simulink model "torqueBalancingSOTSOT2015b86"  (Simulink 8.6)
settings: Solver=FixedStepDiscrete  StartTime=0.0  StopTime="CONFIG.SIMULATION_TIME "  FixedStep=CONFIG.Ts  RelTol=1e-3
InitFcn:
  | cd(fileparts(which(bdroot)));
  | initTorqueBalancingSOT;
undefined symbols (not defined in the file or in its folder): CONFIG, ConstraintsFeetMatrix, gain, references, ROBOT_DOF, ROBOT_DOF_FOR_SIMULINK, sat, SM, sm, upperBoundFeetConstraints, WBT_robotName
libraries: WBToolboxLibrary x135, simulink x8
(part 1 of 3)
settings Model: Creator=daniele  LastModifiedBy=marie
settings DataIOCC: SignalLoggingSaveFormat=Dataset
settings DebuggingCC: FcnCallInpInsideContextMsg=EnableAllAsWarning
settings SFSimCC: SimParseCustomCode=off

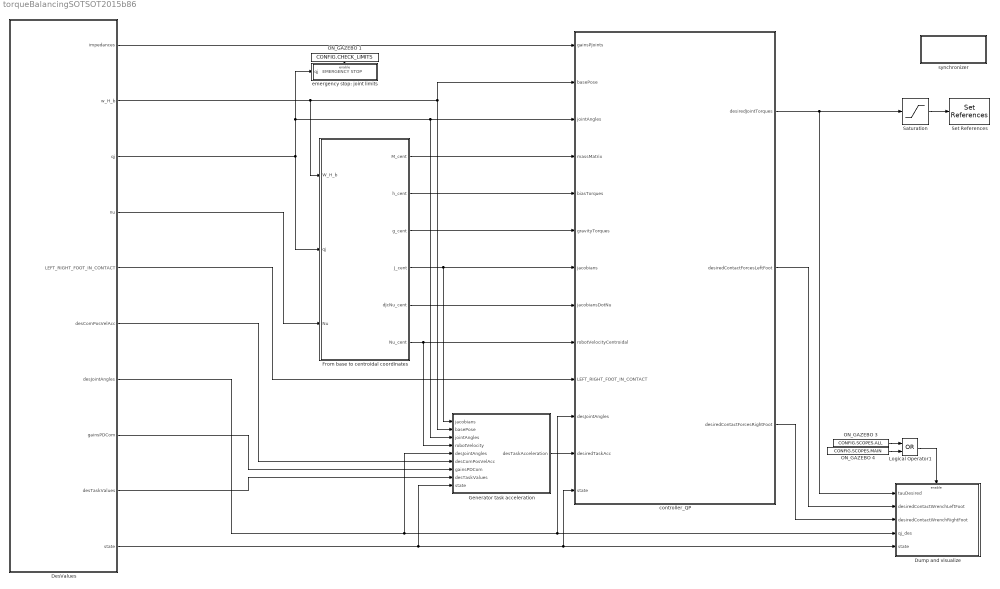
== system torqueBalancingSOTSOT2015b86 ==
  DesValues : Subsystem  Priority=-10
  Dump and visualize : Subsystem
  From base to centroidal coordinates : Subsystem
  Generator task acceleration : Subsystem
  Logical Operator1 : Logic  Operator=OR  AllPortsSameDT=off  OutDataTypeStr=boolean
  ON_GAZEBO 1 : Constant  Value=CONFIG.CHECK_LIMITS
  ON_GAZEBO 3 : Constant  Value=CONFIG.SCOPES.ALL
  ON_GAZEBO 4 : Constant  Value=CONFIG.SCOPES.MAIN
  Saturation : Saturate  UpperLimit=sat.torque  LowerLimit=-sat.torque
  Set References : WBToolboxLibrary/wholeBodyActuators/Set References  controlType=Torque  fullOrSubControl=Full  controlledJoints=''  robotName=WBT_robotName  localName=WBT_modelName  wbiFile=WBT_wbiFilename  wbiList=WBT_wbiList
  controller_QP : Subsystem
  emergency stop: joint limits : Subsystem
  synchronizer : Subsystem
      mask Display: disp('SYNCHRONIZER')
  wires:
  From base to centroidal coordinates/1(M_cent) -> controller_QP/4(massMatrix)
  From base to centroidal coordinates/2(h_cent) -> controller_QP/5(biasTorques)
  controller_QP/1(desiredJointTorques) -> Dump and visualize/1(tauDesired), Saturation/1
  DesValues/7(desJointAngles) -> Dump and visualize/4(qj_des), controller_QP/11(desJointAngles), Generator task acceleration/5(desJointAngles)
  DesValues/5(LEFT_RIGHT_FOOT_IN_CONTACT) -> controller_QP/10(LEFT_RIGHT_FOOT_IN_CONTACT)
  DesValues/6(desComPosVelAcc) -> Generator task acceleration/6(desComPosVelAcc)
  DesValues/1(impedances) -> controller_QP/1(gainsPJoints)
  Saturation/1 -> Set References/1
  DesValues/2(w_H_b) -> From base to centroidal coordinates/1(W_H_b), Generator task acceleration/2(basePose), controller_QP/2(basePose)
  DesValues/4(nu) -> From base to centroidal coordinates/3(Nu)
  Logical Operator1/1 -> Dump and visualize/Enable
  DesValues/10(state) -> Generator task acceleration/9(state), controller_QP/13("state "), Dump and visualize/5(state)
  ON_GAZEBO 1/1 -> emergency stop: joint limits/Enable
  ON_GAZEBO 3/1 -> Logical Operator1/1
  ON_GAZEBO 4/1 -> Logical Operator1/2
  DesValues/3(qj) -> From base to centroidal coordinates/2(qj), emergency stop: joint limits/1(qj   EMERGENCY STOP), Generator task acceleration/3(jointAngles), controller_QP/3(jointAngles)
  From base to centroidal coordinates/3(g_cent) -> controller_QP/6(gravityTorques)
  From base to centroidal coordinates/4(J_cent) -> Generator task acceleration/1(jacobians), controller_QP/7("jacobians ")
  From base to centroidal coordinates/5(dJcNu_cent) -> controller_QP/8(jacobiansDotNu)
  From base to centroidal coordinates/6(Nu_cent) -> Generator task acceleration/4(robotVelocity), controller_QP/9(robotVelocityCentroidal)
  Generator task acceleration/1(desTaskAcceleration) -> controller_QP/12(desiredTaskAcc)
  controller_QP/2(desiredContactForcesLeftFoot) -> Dump and visualize/2(desiredContactWrenchLeftFoot)
  controller_QP/3(desiredContactForcesRightFoot) -> Dump and visualize/3(desiredContactWrenchRightFoot)
  DesValues/8(gainsPDCom) -> Generator task acceleration/7(gainsPDCom)
  DesValues/9(desTaskValues) -> Generator task acceleration/8(desTaskValues)

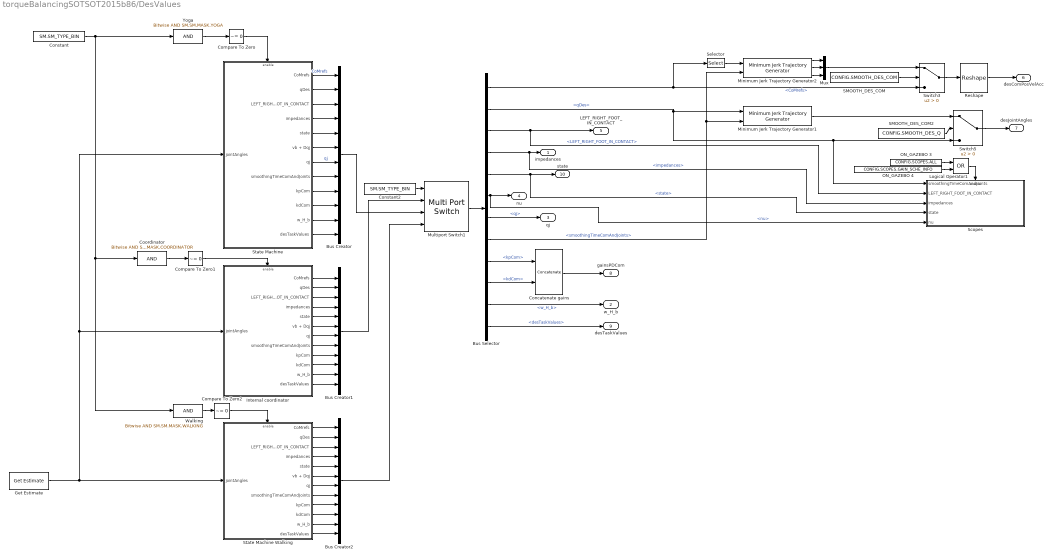
== system torqueBalancingSOTSOT2015b86/DesValues ==
  Bus Creator : BusCreator  Inputs='CoMrefs','qDes','LEFT_RIGHT_FOOT_IN_CONTACT','impedances','state','nu','qj','smoothingTimeComAndJoints','kpCom','kdCom','w_H_b','desTaskValues'
  Bus Creator1 : BusCreator  Inputs='CoMrefs','qDes','LEFT_RIGHT_FOOT_IN_CONTACT','impedances','state','nu','qj','smoothingTimeComAndJoints','kpCom','kdCom','w_H_b','desTaskValues'
  Bus Creator2 : BusCreator  Inputs='CoMrefs','qDes','LEFT_RIGHT_FOOT_IN_CONTACT','impedances','state','nu','qj','smoothingTimeComAndJoints','kpCom','kdCom','w_H_b','desTaskValues'
  Bus Selector : BusSelector  OutputSignals=CoMrefs,qDes,LEFT_RIGHT_FOOT_IN_CONTACT,impedances,state,nu,qj,smoothingTimeComAndJoints,kpCom,kdCom,w_H_b,desTaskValues
  Compare To Zero : simulink/Logic and Bit Operations/Compare To Zero  relop=~=  OutDataTypeStr=boolean
  Compare To Zero1 : simulink/Logic and Bit Operations/Compare To Zero  relop=~=  OutDataTypeStr=boolean
  Compare To Zero2 : simulink/Logic and Bit Operations/Compare To Zero  relop=~=  OutDataTypeStr=boolean
  Concatenate gains : Concatenate  Mode=Multidimensional array  ConcatenateDimension=2
  Constant : Constant  Priority=-10  Value=SM.SM_TYPE_BIN  OutDataTypeStr=uint8
  Constant2 : Constant  Priority=-10  Value=SM.SM_TYPE_BIN  OutDataTypeStr=uint8
  Coordinator : simulink/Logic and Bit Operations/Bitwise Operator  logicop=AND  UseBitMask=on  BitMask=SM.SM.MASK.COORDINATOR  BitMaskRealWorld=Stored Integer
  Get Estimate : WBToolboxLibrary/wholeBodyStates/Get Estimate  estimateType=Joints Position  robotName=WBT_robotName  localName=WBT_modelName  wbiFile=WBT_wbiFilename  wbiList=WBT_wbiList
  Internal coordinator : Subsystem
  Logical Operator1 : Logic  Operator=OR  AllPortsSameDT=off  OutDataTypeStr=boolean
  Minimum Jerk Trajectory Generator1 : WBToolboxLibrary/Utilities/Minimum Jerk Trajectory Generator  externalSettlingTime=on  settlingTime=1  sampleTime=CONFIG.Ts  resetOnSettlingTime=off  firstDerivatives=off  secondDerivatives=off  explicitInitialValue=off
  Minimum Jerk Trajectory Generator2 : WBToolboxLibrary/Utilities/Minimum Jerk Trajectory Generator  externalSettlingTime=on  settlingTime=references.com.smoothingTime  sampleTime=CONFIG.Ts  resetOnSettlingTime=off  firstDerivatives=on  secondDerivatives=on  explicitInitialValue=off
  Multiport Switch1 : MultiPortSwitch  DataPortOrder=Specify indices  DataPortIndices={1, 2, 4}
  Mux : Mux  Inputs=3
  ON_GAZEBO 3 : Constant  Value=CONFIG.SCOPES.ALL
  ON_GAZEBO 4 : Constant  Value=CONFIG.SCOPES.GAIN_SCHE_INFO
  Reshape : Reshape  OutputDimensionality=Customize  OutputDimensions=[3,3]
  SMOOTH_DES_COM : Constant  Value=CONFIG.SMOOTH_DES_COM
  SMOOTH_DES_COM2 : Constant  Value=CONFIG.SMOOTH_DES_Q
  "Scopes  " : Subsystem
  Selector : Selector  InputPortWidth=9  IndexOptions=Index vector (dialog)  Indices=[1 2 3]  OutputSizes=1
  State Machine : Subsystem  Priority=-100
  State Machine Walking : Subsystem  Priority=-100
  Switch3 : Switch  Criteria=u2 > Threshold
  Switch5 : Switch  Criteria=u2 > Threshold
  Walking : simulink/Logic and Bit Operations/Bitwise Operator  logicop=AND  UseBitMask=on  BitMask=SM.SM.MASK.WALKING  BitMaskRealWorld=Stored Integer
  Yoga : simulink/Logic and Bit Operations/Bitwise Operator  logicop=AND  UseBitMask=on  BitMask=SM.SM.MASK.YOGA  BitMaskRealWorld=Stored Integer
  impedances : Outport
  w_H_b : Outport  Port=2
  qj : Outport  Port=3
  nu : Outport  Port=4
  LEFT_RIGHT_FOOT_IN_CONTACT : Outport  Port=5
  desComPosVelAcc : Outport  Port=6
  desJointAngles : Outport  Port=7
  gainsPDCom : Outport  Port=8
  desTaskValues : Outport  Port=9
  state : Outport  Port=10
  wires:
  Reshape/1 -> desComPosVelAcc/1
  Minimum Jerk Trajectory Generator2/1 -> Mux/1
  Minimum Jerk Trajectory Generator2/2 -> Mux/2
  Minimum Jerk Trajectory Generator2/3 -> Mux/3
  Switch3/1 -> Reshape/1
  SMOOTH_DES_COM/1 -> Switch3/2
  SMOOTH_DES_COM2/1 -> Switch5/2
  Switch5/1 -> desJointAngles/1
  State Machine/3(LEFT_RIGHT_FOOT_IN_CONTACT) -> Bus Creator/3
  State Machine/2(qDes) -> Bus Creator/2
  State Machine/1(CoMrefs) -> Bus Creator/1  "CoMrefs"
  State Machine/4(impedances) -> Bus Creator/4
  State Machine/5(state) -> Bus Creator/5
  State Machine/6(vb + Dqj) -> Bus Creator/6
  State Machine/7(qj) -> Bus Creator/7  "qj"
  Bus Selector/7 -> qj/1  "<qj>"
  Yoga/1 -> Compare To Zero/1
  Walking/1 -> Compare To Zero2/1
  Compare To Zero/1 -> State Machine/Enable
  Compare To Zero2/1 -> State Machine Walking/Enable
  Bus Selector/11 -> w_H_b/1  "<w_H_b>"
  Bus Selector/5 -> "Scopes  "/4(state), state/1  "<state>"
  State Machine/8(smoothingTimeComAndJoints) -> Bus Creator/8
  Bus Selector/8 -> Minimum Jerk Trajectory Generator2/2, Minimum Jerk Trajectory Generator1/2  "<smoothingTimeComAndJoints>"
  Logical Operator1/1 -> "Scopes  "/Enable
  Bus Selector/1 -> Selector/1, Switch3/3  "<CoMrefs>"
  Mux/1 -> Switch3/1
  Selector/1 -> Minimum Jerk Trajectory Generator2/1
  Bus Selector/2 -> Minimum Jerk Trajectory Generator1/1, "Scopes  "/1(smoothingTimeComAndJoints), Switch5/3  "<qDes>"
  Minimum Jerk Trajectory Generator1/1 -> Switch5/1
  ON_GAZEBO 3/1 -> Logical Operator1/1
  ON_GAZEBO 4/1 -> Logical Operator1/2
  Bus Selector/6 -> nu/1, "Scopes  "/5(nu)  "<nu>"
  State Machine/9(kpCom) -> Bus Creator/9
  State Machine/10(kdCom) -> Bus Creator/10
  Multiport Switch1/1 -> Bus Selector/1
  Bus Selector/4 -> "Scopes  "/3(impedances), impedances/1  "<impedances>"
  Bus Selector/3 -> "Scopes  "/2(LEFT_RIGHT_FOOT_IN_CONTACT), LEFT_RIGHT_FOOT_IN_CONTACT/1  "<LEFT_RIGHT_FOOT_IN_CONTACT>"
  Constant2/1 -> Multiport Switch1/1
  Concatenate gains/1 -> gainsPDCom/1
  Bus Selector/9 -> Concatenate gains/1  "<kpCom>"
  Bus Selector/10 -> Concatenate gains/2  "<kdCom>"
  Constant/1 -> Walking/1, Coordinator/1, Yoga/1
  Coordinator/1 -> Compare To Zero1/1
  Compare To Zero1/1 -> Internal coordinator/Enable
  Get Estimate/1 -> State Machine Walking/1(jointAngles), State Machine/1(jointAngles), Internal coordinator/1(jointAngles)
  State Machine/11(w_H_b) -> Bus Creator/11
  Bus Creator/1 -> Multiport Switch1/3
  Internal coordinator/1(CoMrefs) -> Bus Creator1/1
  Internal coordinator/2(qDes) -> Bus Creator1/2
  Internal coordinator/3(LEFT_RIGHT_FOOT_IN_CONTACT) -> Bus Creator1/3
  Internal coordinator/4(impedances) -> Bus Creator1/4
  Internal coordinator/5(state) -> Bus Creator1/5
  Internal coordinator/6(vb + Dqj) -> Bus Creator1/6
  Internal coordinator/7(qj) -> Bus Creator1/7
  Internal coordinator/8(smoothingTimeComAndJoints) -> Bus Creator1/8
  Internal coordinator/9(kpCom) -> Bus Creator1/9
  Internal coordinator/10(kdCom) -> Bus Creator1/10
  Internal coordinator/11(w_H_b) -> Bus Creator1/11
  State Machine Walking/1(CoMrefs) -> Bus Creator2/1
  State Machine Walking/2(qDes) -> Bus Creator2/2
  State Machine Walking/3(LEFT_RIGHT_FOOT_IN_CONTACT) -> Bus Creator2/3
  State Machine Walking/4(impedances) -> Bus Creator2/4
  State Machine Walking/5(state) -> Bus Creator2/5
  State Machine Walking/6(vb + Dqj) -> Bus Creator2/6
  State Machine Walking/8(smoothingTimeComAndJoints) -> Bus Creator2/8
  State Machine Walking/9(kpCom) -> Bus Creator2/9
  State Machine Walking/10(kdCom) -> Bus Creator2/10
  State Machine Walking/11(w_H_b) -> Bus Creator2/11
  Bus Creator2/1 -> Multiport Switch1/4
  Bus Creator1/1 -> Multiport Switch1/2
  State Machine/12(desTaskValues) -> Bus Creator/12
  Internal coordinator/12(desTaskValues) -> Bus Creator1/12
  State Machine Walking/12(desTaskValues) -> Bus Creator2/12
  Bus Selector/12 -> desTaskValues/1  "<desTaskValues>"
  State Machine Walking/7(qj) -> Bus Creator2/7

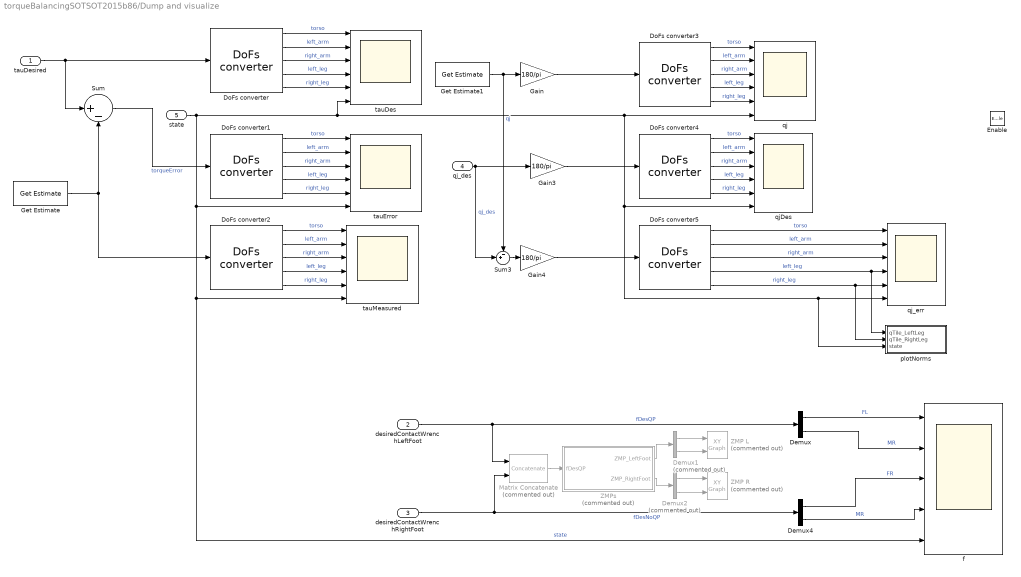
== system torqueBalancingSOTSOT2015b86/Dump and visualize ==
  tauDesired : Inport
  desiredContactWrenchLeftFoot : Inport  Port=2
  desiredContactWrenchRightFoot : Inport  Port=3
  qj_des : Inport  Port=4
  state : Inport  Port=5
  Enable : EnablePort
  Demux : Demux  Outputs=2
  Demux1 : Demux  Commented=on  Outputs=2
  Demux2 : Demux  Commented=on  Outputs=2
  Demux4 : Demux  Outputs=2
  DoFs converter{,1..5} (6 alike) : WBToolboxLibrary/Utilities/DoFs converter  yarp2WBIOption=From WBI to YARP  robotName=WBT_robotName  localName=WBT_modelName  wbiFile=WBT_wbiFilename  wbiList=WBT_wbiList
  Gain : Gain  Gain=180/pi
  Gain3 : Gain  Gain=180/pi
  Gain4 : Gain  Gain=180/pi
  Get Estimate : WBToolboxLibrary/wholeBodyStates/Get Estimate  estimateType=Joints Torque  robotName=WBT_robotName  localName=WBT_modelName  wbiFile=WBT_wbiFilename  wbiList=WBT_wbiList
  Get Estimate1 : WBToolboxLibrary/wholeBodyStates/Get Estimate  estimateType=Joints Position  robotName=WBT_robotName  localName=WBT_modelName  wbiFile=WBT_wbiFilename  wbiList=WBT_wbiList
  Matrix Concatenate : Concatenate  Commented=on  Mode=Multidimensional array
  Sum : Sum  Inputs=|+-
  Sum3 : Sum  Inputs=-+|
  ZMP L : simulink/Sinks/XY Graph  Commented=on  xmin=gain.footSize(1,1)  xmax=gain.footSize(1,2)  ymin=gain.footSize(2,1)  ymax=gain.footSize(2,2)  st=-1
  ZMP R : simulink/Sinks/XY Graph  Commented=on  xmin=gain.footSize(1,1)  xmax=gain.footSize(1,2)  ymin=gain.footSize(2,1)  ymax=gain.footSize(2,2)  st=-1
  ZMPs : Subsystem  Commented=on
  f : Scope  NumInputPorts=5
  plotNorms : Subsystem
  qj : Scope  NumInputPorts=6
  qjDes : Scope  NumInputPorts=6
  qj_err : Scope  NumInputPorts=6
  tauDes : Scope  NumInputPorts=6
  tauError : Scope  NumInputPorts=6
  tauMeasured : Scope  NumInputPorts=6
  wires:
  Get Estimate1/1 -> Sum3/1, Gain/1  "qj"
  Gain/1 -> DoFs converter3/1
  DoFs converter3/5 -> qj/5  "right_leg"
  DoFs converter3/1 -> qj/1  "torso"
  DoFs converter3/2 -> qj/2  "left_arm"
  DoFs converter3/4 -> qj/4  "left_leg"
  DoFs converter3/3 -> qj/3  "right_arm"
  desiredContactWrenchLeftFoot/1 -> Matrix Concatenate/1, Demux/1  "fDesQP"
  ZMPs/1(ZMP_LeftFoot) -> Demux1/1
  ZMPs/2(ZMP_RightFoot) -> Demux2/1
  Demux1/1 -> ZMP L/1
  Demux1/2 -> ZMP L/2
  Demux2/1 -> ZMP R/1
  Demux2/2 -> ZMP R/2
  desiredContactWrenchRightFoot/1 -> Matrix Concatenate/2, Demux4/1  "fDesNoQP"
  tauDesired/1 -> DoFs converter/1, Sum/1
  Get Estimate/1 -> DoFs converter2/1, Sum/2
  DoFs converter/5 -> tauDes/5  "right_leg"
  DoFs converter/1 -> tauDes/1  "torso"
  DoFs converter/2 -> tauDes/2  "left_arm"
  DoFs converter/4 -> tauDes/4  "left_leg"
  DoFs converter/3 -> tauDes/3  "right_arm"
  DoFs converter1/5 -> tauError/5  "right_leg"
  DoFs converter1/1 -> tauError/1  "torso"
  DoFs converter1/2 -> tauError/2  "left_arm"
  DoFs converter1/4 -> tauError/4  "left_leg"
  DoFs converter1/3 -> tauError/3  "right_arm"
  Sum/1 -> DoFs converter1/1  "torqueError"
  DoFs converter2/5 -> tauMeasured/5  "right_leg"
  DoFs converter2/1 -> tauMeasured/1  "torso"
  DoFs converter2/2 -> tauMeasured/2  "left_arm"
  DoFs converter2/4 -> tauMeasured/4  "left_leg"
  DoFs converter2/3 -> tauMeasured/3  "right_arm"
  qj_des/1 -> Sum3/2, Gain3/1  "qj_des"
  Gain3/1 -> DoFs converter4/1
  DoFs converter4/5 -> qjDes/5  "right_leg"
  DoFs converter4/1 -> qjDes/1  "torso"
  DoFs converter4/2 -> qjDes/2  "left_arm"
  DoFs converter4/4 -> qjDes/4  "left_leg"
  DoFs converter4/3 -> qjDes/3  "right_arm"
  Gain4/1 -> DoFs converter5/1
  DoFs converter5/5 -> plotNorms/2(qTile_RightLeg), qj_err/5  "right_leg"
  DoFs converter5/1 -> qj_err/1  "torso"
  DoFs converter5/2 -> qj_err/2  "left_arm"
  DoFs converter5/4 -> plotNorms/1(qTile_LeftLeg), qj_err/4  "left_leg"
  DoFs converter5/3 -> qj_err/3  "right_arm"
  Sum3/1 -> Gain4/1
  state/1 -> tauDes/6, plotNorms/3(state), qj_err/6, qjDes/6, qj/6, f/5, tauMeasured/6, tauError/6  "state"
  Demux/1 -> f/1  "FL"
  Demux/2 -> f/2  "MR"
  Demux4/1 -> f/3  "FR"
  Demux4/2 -> f/4  "MR"
  Matrix Concatenate/1 -> ZMPs/1(fDesQP)

== system torqueBalancingSOTSOT2015b86/From base to centroidal coordinates ==
  W_H_b : Inport
  qj : Inport  Port=2
  Nu : Inport  Port=3
  Centroidal tranformation : Subsystem
  CoM and Base Kinematics : Subsystem
  Jacobians : Subsystem
  Switch{1..6} (6 alike) : Switch  Criteria=u2 > Threshold
  System Dynamics : Subsystem
  USE_IMU4EST_BASE{,1..5} (6 alike) : Constant  Value=CONFIG.USE_CENTROIDALDYN
  M_cent : Outport
  h_cent : Outport  Port=2
  g_cent : Outport  Port=3
  J_cent : Outport  Port=4
  dJcNu_cent : Outport  Port=5
  Nu_cent : Outport  Port=6
  wires:
  Jacobians/2(dJNu) -> Switch4/3, Centroidal tranformation/10(dJcNu)
  System Dynamics/1(h) -> Switch1/3, Centroidal tranformation/2(h)
  System Dynamics/2(g) -> Switch2/3, Centroidal tranformation/3(g)
  System Dynamics/3(M) -> Switch6/3, Centroidal tranformation/4(M)
  CoM and Base Kinematics/1(dx_b) -> Centroidal tranformation/6(dx_b)
  CoM and Base Kinematics/2(xCoM) -> Centroidal tranformation/7(xCoM)
  CoM and Base Kinematics/3(dxCoM) -> Centroidal tranformation/8(dxCoM)
  Jacobians/1(J) -> Switch3/3, Centroidal tranformation/9(Jc)
  qj/1 -> CoM and Base Kinematics/2(qj), System Dynamics/2(qj), Jacobians/2(qj)
  Nu/1 -> Jacobians/3(Nu), CoM and Base Kinematics/3(Nu), Switch5/3, Centroidal tranformation/5(Nu), System Dynamics/3(Nu)
  W_H_b/1 -> Centroidal tranformation/1(w_H_b), Jacobians/1(W_H_b), System Dynamics/1(W_H_b), CoM and Base Kinematics/1(W_H_b)
  USE_IMU4EST_BASE/1 -> Switch6/2
  Switch6/1 -> M_cent/1
  Centroidal tranformation/1(M_centr) -> Switch6/1
  USE_IMU4EST_BASE1/1 -> Switch1/2
  USE_IMU4EST_BASE2/1 -> Switch2/2
  USE_IMU4EST_BASE3/1 -> Switch3/2
  USE_IMU4EST_BASE4/1 -> Switch4/2
  USE_IMU4EST_BASE5/1 -> Switch5/2
  Centroidal tranformation/2(h_centr) -> Switch1/1
  Switch1/1 -> h_cent/1
  Centroidal tranformation/3(g_centr) -> Switch2/1
  Centroidal tranformation/4(Jc_centr) -> Switch3/1
  Switch2/1 -> g_cent/1
  Switch3/1 -> J_cent/1
  Centroidal tranformation/5(dJcNu_centr) -> Switch4/1
  Switch4/1 -> dJcNu_cent/1
  Switch5/1 -> Nu_cent/1
  Centroidal tranformation/6(Nu_centr) -> Switch5/1

== system torqueBalancingSOTSOT2015b86/Generator task acceleration ==
  jacobians : Inport
  basePose : Inport  Port=2
  jointAngles : Inport  Port=3
  robotVelocity : Inport  Port=4
  desJointAngles : Inport  Port=5
  desComPosVelAcc : Inport  Port=6
  gainsPDCom : Inport  Port=7
  desTaskValues : Inport  Port=8
  state : Inport  Port=9
  Bus Selector : BusSelector  OutputSignals=desRootRotPosVelAcc,desLFootRotPosVelAcc,desLFootOriginPosVelAcc,desRFootRotPosVelAcc,desRFootOriginPosVelAcc
  Dump and visualize : Subsystem
  Logical Operator1 : Logic  Operator=OR  AllPortsSameDT=off  OutDataTypeStr=boolean
  ON_GAZEBO 3 : Constant  Value=CONFIG.SCOPES.ALL
  ON_GAZEBO 4 : Constant  Value=CONFIG.SCOPES.MAIN
  Product : Product  Multiplication=Matrix(*)
  desiredTaskAcceleration : MATLAB Function  TreatAsAtomicUnit=on
      settings: PermitHierarchicalResolution=ParametersOnly
  fromDesiredJointAngles to  desRootRotPosVelAcc3 : Subsystem
  leftFootPose : WBToolboxLibrary/wholeBodyModel/Kinematics/Forward Kinematics  frameName='l_sole'  robotName=WBT_robotName  localName=WBT_modelName  wbiFile=WBT_wbiFilename  wbiList=WBT_wbiList
  rightFootPose : WBToolboxLibrary/wholeBodyModel/Kinematics/Forward Kinematics  frameName='r_sole'  robotName=WBT_robotName  localName=WBT_modelName  wbiFile=WBT_wbiFilename  wbiList=WBT_wbiList
  xCom : Subsystem
  desTaskAcceleration : Outport
  wires:
  desiredTaskAcceleration/1(desiredTaskAcc) -> desTaskAcceleration/1
  jointAngles/1 -> rightFootPose/2, leftFootPose/2, xCom/2(qj)
  robotVelocity/1 -> Product/2
  basePose/1 -> rightFootPose/1, leftFootPose/1, xCom/1(w_H_b)
  jacobians/1 -> Product/1
  desJointAngles/1 -> fromDesiredJointAngles to  desRootRotPosVelAcc3/1(desJointAngles)
  xCom/1(xCom) -> desiredTaskAcceleration/1(comPos)
  fromDesiredJointAngles to  desRootRotPosVelAcc3/1(fixed_link_R_root) -> desiredTaskAcceleration/3(w_R_root)
  desComPosVelAcc/1 -> desiredTaskAcceleration/2(desComPosVelAcc), Dump and visualize/3(comDes)
  leftFootPose/1 -> desiredTaskAcceleration/5(w_H_l_sole)
  Bus Selector/2 -> Dump and visualize/8(desLFootRot), desiredTaskAcceleration/6(desLFootRotPosVelAcc)  "<desLFootRotPosVelAcc>"
  Product/1 -> desiredTaskAcceleration/11(taskVelocities)
  gainsPDCom/1 -> desiredTaskAcceleration/12(gainsPDCom)
  Bus Selector/1 -> desiredTaskAcceleration/4(desRootRotPosVelAcc), Dump and visualize/1(desRootRot)  "<desRootRotPosVelAcc>"
  Bus Selector/3 -> desiredTaskAcceleration/7(desLFootOriginPosVelAcc), Dump and visualize/6(desLFootPos)  "<desLFootOriginPosVelAcc>"
  rightFootPose/1 -> desiredTaskAcceleration/8(w_H_r_sole)
  Bus Selector/4 -> desiredTaskAcceleration/9(desRFootRotPosVelAcc), Dump and visualize/12(desRFootRot)  "<desRFootRotPosVelAcc>"
  Bus Selector/5 -> desiredTaskAcceleration/10(desRFootOriginPosVelAcc), Dump and visualize/10(desRFootPos)  "<desRFootOriginPosVelAcc>"
  Logical Operator1/1 -> Dump and visualize/Enable
  ON_GAZEBO 3/1 -> Logical Operator1/1
  ON_GAZEBO 4/1 -> Logical Operator1/2
  desiredTaskAcceleration/2(comError) -> Dump and visualize/2(comErr)
  desiredTaskAcceleration/3(rootRotErr) -> Dump and visualize/4(rootRotErr)
  desiredTaskAcceleration/4(lFootPosErr) -> Dump and visualize/5(lFootPosErr)
  desiredTaskAcceleration/5(lFootRotErr) -> Dump and visualize/7(lFoorRotErr)
  desiredTaskAcceleration/6(rFootPosErr) -> Dump and visualize/9(rFootPosErr)
  desiredTaskAcceleration/7(rFootRotErr) -> Dump and visualize/11(rFoorRotErr)
  state/1 -> Dump and visualize/13(state), fromDesiredJointAngles to  desRootRotPosVelAcc3/2(state)
  desTaskValues/1 -> Bus Selector/1

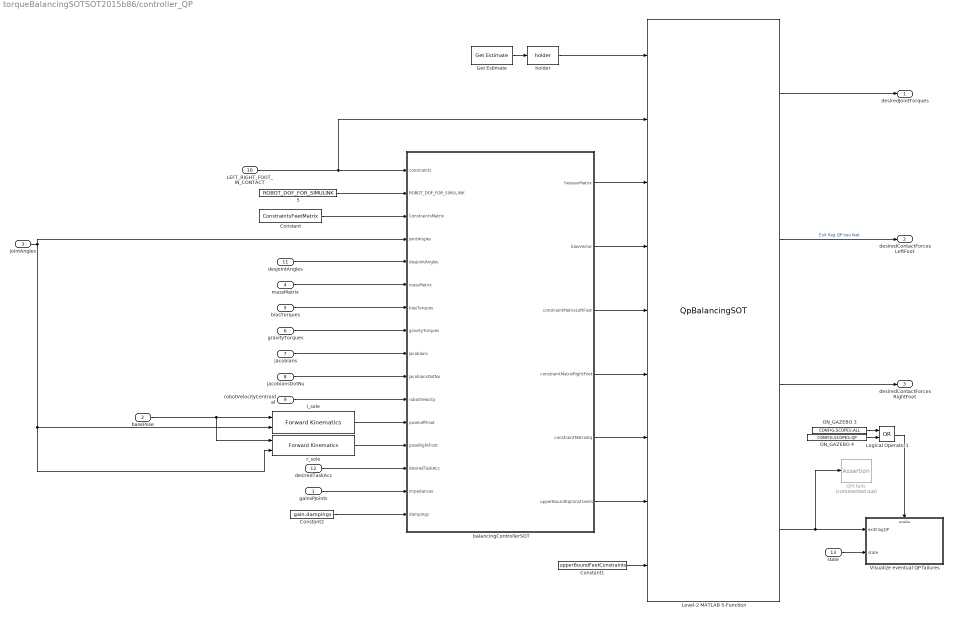
== system torqueBalancingSOTSOT2015b86/controller_QP ==
  gainsPJoints : Inport
  basePose : Inport  Port=2
  jointAngles : Inport  Port=3
  massMatrix : Inport  Port=4
  biasTorques : Inport  Port=5
  gravityTorques : Inport  Port=6
  "jacobians " : Inport  Port=7
  jacobiansDotNu : Inport  Port=8
  robotVelocityCentroidal : Inport  Port=9
  LEFT_RIGHT_FOOT_IN_CONTACT : Inport  Port=10
  desJointAngles : Inport  Port=11
  desiredTaskAcc : Inport  Port=12
  "state " : Inport  Port=13
  "    5" : Constant  Value=ROBOT_DOF_FOR_SIMULINK
  Constant : Constant  Value=ConstraintsFeetMatrix
  Constant1 : Constant  Value=upperBoundFeetConstraints
  Constant2 : Constant  Value=gain.dampings
  Get Estimate : WBToolboxLibrary/wholeBodyStates/Get Estimate  estimateType=Joints Torque  robotName=WBT_robotName  localName=WBT_modelName  wbiFile=WBT_wbiFilename  wbiList=WBT_wbiList
  Level-2 MATLAB S-Function : M-S-Function  FunctionName=QpBalancingSOT  Parameters=ROBOT_DOF,sat.torqueDot,CONFIG.Ts,CONFIG.QP.USE_CONTINUITY_CONSTRAINTS,CONFIG.QP.USE_STRICT_TASK_PRIORITIES  mask{robotDofs=ROBOT_DOF, tauDotMax=sat.torqueDot, Ts=CONFIG.Ts}
      mask prompts: robotDofs "Robt degrees of freedom"; tauDotMax "Maximum derivative of torques"; Ts "Controller period"
      mask Display: disp('QP')
  Logical Operator1 : Logic  Operator=OR  AllPortsSameDT=off  OutDataTypeStr=boolean
  ON_GAZEBO 3 : Constant  Value=CONFIG.SCOPES.ALL
  ON_GAZEBO 4 : Constant  Value=CONFIG.SCOPES.QP
  QPt fails : Assertion  Commented=on
  Visualize eventual QP failures : Subsystem
  balancingControllerSOT : MATLAB Function  TreatAsAtomicUnit=on
      settings: PermitHierarchicalResolution=ParametersOnly
  "holder " : WBToolboxLibrary/Utilities/holder 
  l_sole : WBToolboxLibrary/wholeBodyModel/Kinematics/Forward Kinematics  frameName='l_sole'  robotName=WBT_robotName  localName=WBT_modelName  wbiFile=WBT_wbiFilename  wbiList=WBT_wbiList
  r_sole : WBToolboxLibrary/wholeBodyModel/Kinematics/Forward Kinematics  frameName='r_sole'  robotName=WBT_robotName  localName=WBT_modelName  wbiFile=WBT_wbiFilename  wbiList=WBT_wbiList
  desiredJointTorques : Outport
  desiredContactForcesLeftFoot : Outport  Port=2
  desiredContactForcesRightFoot : Outport  Port=3
  wires:
  jointAngles/1 -> r_sole/2, l_sole/2, balancingControllerSOT/4(jointAngles)
  desJointAngles/1 -> balancingControllerSOT/5(desJointAngles)
  gainsPJoints/1 -> balancingControllerSOT/15(impedances)
  "    5"/1 -> balancingControllerSOT/2(ROBOT_DOF_FOR_SIMULINK)
  Constant/1 -> balancingControllerSOT/3(ConstraintsMatrix)
  Constant1/1 -> Level-2 MATLAB S-Function/9
  basePose/1 -> r_sole/1, l_sole/1
  desiredTaskAcc/1 -> balancingControllerSOT/14(desiredTaskAcc)
  r_sole/1 -> balancingControllerSOT/13(poseRightFoot)
  l_sole/1 -> balancingControllerSOT/12(poseLeftFoot)
  robotVelocityCentroidal/1 -> balancingControllerSOT/11(robotVelocity)
  gravityTorques/1 -> balancingControllerSOT/8(gravityTorques)
  biasTorques/1 -> balancingControllerSOT/7(biasTorques)
  massMatrix/1 -> balancingControllerSOT/6(massMatrix)
  Logical Operator1/1 -> Visualize eventual QP failures/Enable
  LEFT_RIGHT_FOOT_IN_CONTACT/1 -> Level-2 MATLAB S-Function/2, balancingControllerSOT/1(constraints)
  ON_GAZEBO 3/1 -> Logical Operator1/1
  ON_GAZEBO 4/1 -> Logical Operator1/2
  balancingControllerSOT/1(hessianMatrix) -> Level-2 MATLAB S-Function/3
  balancingControllerSOT/2(biasVector) -> Level-2 MATLAB S-Function/4
  balancingControllerSOT/3(constraintMatrixLeftFoot) -> Level-2 MATLAB S-Function/5
  balancingControllerSOT/4(constraintMatrixRightFoot) -> Level-2 MATLAB S-Function/6
  "jacobians "/1 -> balancingControllerSOT/9(jacobians)
  jacobiansDotNu/1 -> balancingControllerSOT/10(jacobiansDotNu)
  Level-2 MATLAB S-Function/1 -> desiredJointTorques/1
  balancingControllerSOT/6(upperBoundEqConstraints) -> Level-2 MATLAB S-Function/8
  balancingControllerSOT/5(constraintMatrixEq) -> Level-2 MATLAB S-Function/7
  Level-2 MATLAB S-Function/3 -> desiredContactForcesRightFoot/1
  Level-2 MATLAB S-Function/2 -> desiredContactForcesLeftFoot/1  "Exit flag QP two feet"
  "state "/1 -> Visualize eventual QP failures/2(state)
  Level-2 MATLAB S-Function/4 -> QPt fails/1, Visualize eventual QP failures/1(exitFlagQP)
  Constant2/1 -> balancingControllerSOT/16(dampings)
  Get Estimate/1 -> "holder "/1
  "holder "/1 -> Level-2 MATLAB S-Function/1

== system torqueBalancingSOTSOT2015b86/emergency stop: joint limits ==
  qj   EMERGENCY STOP : Inport
  Enable : EnablePort
  Assertion : Assertion
  Get Limits : WBToolboxLibrary/wholeBodyStates/Get Limits  limitsType=Position  robotName=WBT_robotName  localName=WBT_modelName  wbiFile=WBT_wbiFilename  wbiList=WBT_wbiList
  MATLAB Function : MATLAB Function  TreatAsAtomicUnit=on
      settings: PermitHierarchicalResolution=ParametersOnly
  index1 : Constant  Value=0.01  VectorParams1D=off
  wires:
  Get Limits/1 -> MATLAB Function/1(umin)
  Get Limits/2 -> MATLAB Function/2(umax)
  index1/1 -> MATLAB Function/4(tol)
  qj   EMERGENCY STOP/1 -> MATLAB Function/3(u)
  MATLAB Function/1(inRange) -> Assertion/1

== system torqueBalancingSOTSOT2015b86/synchronizer ==
  GAZEBO_SYNCHRONIZER : Subsystem
  Logical Operator : Logic  Operator=NOT  AllPortsSameDT=off  OutDataTypeStr=boolean
  "ON_GAZEBO " : Constant  Value=CONFIG.ON_GAZEBO
  REAL_TIME_SYNC : Subsystem
  wires:
  Logical Operator/1 -> REAL_TIME_SYNC/Enable
  "ON_GAZEBO "/1 -> GAZEBO_SYNCHRONIZER/Enable, Logical Operator/1

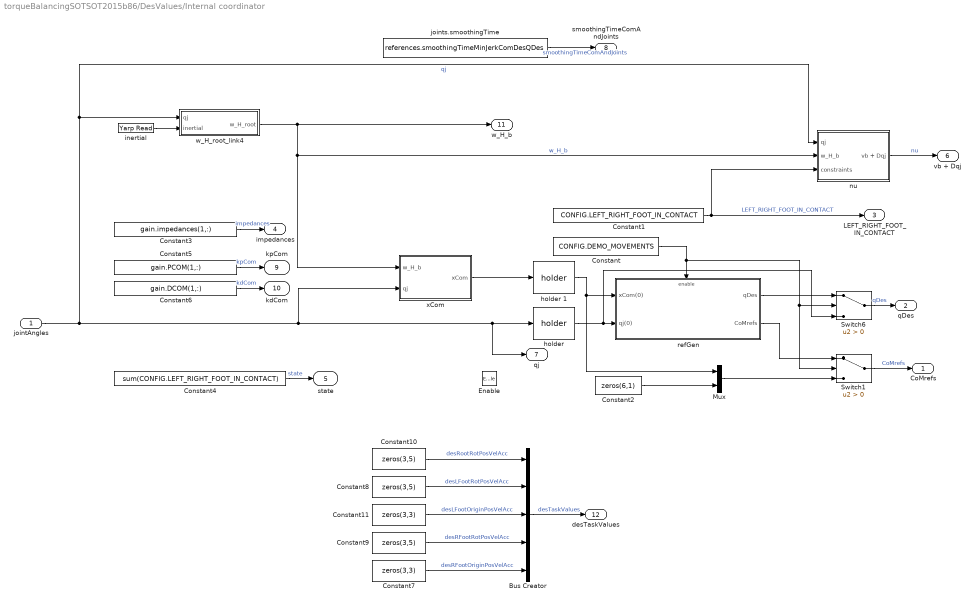
== system torqueBalancingSOTSOT2015b86/DesValues/Internal coordinator ==
  jointAngles : Inport
  Enable : EnablePort
  Bus Creator : BusCreator  Inputs='desRootRotPosVelAcc','desLFootRotPosVelAcc','desLFootOriginPosVelAcc','desRFootRotPosVelAcc','desRFootOriginPosVelAcc'
  Constant : Constant  Value=CONFIG.DEMO_MOVEMENTS
  Constant1 : Constant  Value=CONFIG.LEFT_RIGHT_FOOT_IN_CONTACT
  Constant10 : Constant  Value=zeros(3,5)
  Constant11 : Constant  Value=zeros(3,3)
  Constant2 : Constant  Value=zeros(6,1)
  Constant3 : Constant  Value=gain.impedances(1,:)
  Constant4 : Constant  Value=sum(CONFIG.LEFT_RIGHT_FOOT_IN_CONTACT)
  Constant5 : Constant  Value=gain.PCOM(1,:)
  Constant6 : Constant  Value=gain.DCOM(1,:)
  Constant7 : Constant  Value=zeros(3,3)
  Constant8 : Constant  Value=zeros(3,5)
  Constant9 : Constant  Value=zeros(3,5)
  Mux : Mux  Inputs=2
  Switch1 : Switch  Criteria=u2 > Threshold
  Switch6 : Switch  Criteria=u2 > Threshold
  "holder " : WBToolboxLibrary/Utilities/holder 
  holder 1 : WBToolboxLibrary/Utilities/holder 
  inertial : WBToolboxLibrary/Utilities/Yarp Read  portName=PORTS.IMU  signalSize=12  blocking=off  timestamp=off  autoconnect=on  errorOnConnection=on
  joints.smoothingTime : Constant  Value=references.smoothingTimeMinJerkComDesQDes
  nu : Subsystem
  refGen : Subsystem
  w_H_root_link4 : Subsystem  mask{link_name='l_sole'}
      mask prompts: link_name "link name"
      mask help:
      | This block evaluates the homogeneous transformation between the world and the root link, i.e. ^wH_b. It assumes that the link specified by the variable 'link_name' has a constant position
      | w.r.t. an inertial frame, but it can rotate arbitrarily. This rotation is retrived from the IMU sensor.
      mask Display:
      | str = strrep(link_name, '_','\_');
      | port_label('output',1,['{}^{',str '}H_{root}'],'texmode','on')
      | clear str;
      | 
      | port_label('input',1,'q_j','texmode','on')
      | 
      | port_label('input',2,'inertial','texmode','on')
  xCom : Subsystem
  CoMrefs : Outport
  qDes : Outport  Port=2
  LEFT_RIGHT_FOOT_IN_CONTACT : Outport  Port=3
  impedances : Outport  Port=4
  state : Outport  Port=5
  vb + Dqj : Outport  Port=6
  qj : Outport  Port=7
  smoothingTimeComAndJoints : Outport  Port=8
  kpCom : Outport  Port=9
  kdCom : Outport  Port=10
  w_H_b : Outport  Port=11
  desTaskValues : Outport  Port=12
  wires:
  Constant1/1 -> nu/3("constraints "), LEFT_RIGHT_FOOT_IN_CONTACT/1  "LEFT_RIGHT_FOOT_IN_CONTACT"
  "holder "/1 -> Switch6/3, refGen/2(qj(0))
  Constant/1 -> Switch1/2, Switch6/2, refGen/Enable
  Switch6/1 -> qDes/1  "qDes"
  Switch1/1 -> CoMrefs/1  "CoMrefs"
  refGen/1(qDes) -> Switch6/1
  refGen/2(CoMrefs) -> Switch1/1
  Mux/1 -> Switch1/3
  Constant2/1 -> Mux/2
  Constant3/1 -> impedances/1  "impedances"
  Constant4/1 -> state/1  "state"
  nu/1(vb + Dqj) -> vb + Dqj/1  "nu"
  holder 1/1 -> Mux/1, refGen/1(xCom(0))
  w_H_root_link4/1(w_H_root) -> nu/2(w_H_b), xCom/1(w_H_b), w_H_b/1  "w_H_b"
  xCom/1(xCom) -> holder 1/1
  joints.smoothingTime/1 -> smoothingTimeComAndJoints/1  "smoothingTimeComAndJoints"
  jointAngles/1 -> w_H_root_link4/1(qj), nu/1(qj), xCom/2(qj), "holder "/1, qj/1  "qj"
  inertial/1 -> w_H_root_link4/2(inertial)
  Constant5/1 -> kpCom/1  "kpCom"
  Constant6/1 -> kdCom/1  "kdCom"
  Constant8/1 -> Bus Creator/2  "desLFootRotPosVelAcc"
  Constant9/1 -> Bus Creator/4  "desRFootRotPosVelAcc"
  Constant11/1 -> Bus Creator/3  "desLFootOriginPosVelAcc"
  Constant10/1 -> Bus Creator/1  "desRootRotPosVelAcc"
  Bus Creator/1 -> desTaskValues/1  "desTaskValues"
  Constant7/1 -> Bus Creator/5  "desRFootOriginPosVelAcc"

== system torqueBalancingSOTSOT2015b86/DesValues/Scopes   ==
  smoothingTimeComAndJoints : Inport
  LEFT_RIGHT_FOOT_IN_CONTACT : Inport  Port=2
  impedances : Inport  Port=3
  state : Inport  Port=4
  nu : Inport  Port=5
  Enable : EnablePort
  Demux : Demux  Outputs=2
  DoFs converter : WBToolboxLibrary/Utilities/DoFs converter  yarp2WBIOption=From WBI to YARP  robotName=WBT_robotName  localName=WBT_modelName  wbiFile=WBT_wbiFilename  wbiList=WBT_wbiList
  DoFs converter1 : WBToolboxLibrary/Utilities/DoFs converter  yarp2WBIOption=From WBI to YARP  robotName=WBT_robotName  localName=WBT_modelName  wbiFile=WBT_wbiFilename  wbiList=WBT_wbiList
  Gain : Gain  Gain=180/pi
  Gain1 : Gain  Gain=180/pi
  Impedances(t) : Scope  NumInputPorts=6
  Left right foot in contact : Scope
  Selector1 : Selector  InputPortWidth=6+ROBOT_DOF  IndexOptions=Index vector (dialog)  Indices=[7:6+ROBOT_DOF]  OutputSizes=1
  Selector2 : Selector  InputPortWidth=6+ROBOT_DOF  IndexOptions=Index vector (dialog)  Indices=[1:6]  OutputSizes=1
  jointsSmoothingTime : Scope  NumInputPorts=2
  linear and angular  base velocity : Scope  NumInputPorts=3
  "qjDot(t) " : Scope  NumInputPorts=6
  wires:
  state/1 -> "qjDot(t) "/6, linear and angular  base velocity/3, Impedances(t)/6, jointsSmoothingTime/2  "state"
  LEFT_RIGHT_FOOT_IN_CONTACT/1 -> Left right foot in contact/1  "Left right foot in contact"
  impedances/1 -> DoFs converter/1
  smoothingTimeComAndJoints/1 -> jointsSmoothingTime/1  "smoothingTimeComAndJoints"
  DoFs converter/4 -> Impedances(t)/4  "left_leg"
  DoFs converter/5 -> Impedances(t)/5  "right_leg"
  DoFs converter/3 -> Impedances(t)/3  "right_arm"
  DoFs converter/1 -> Impedances(t)/1  "torso"
  DoFs converter/2 -> Impedances(t)/2  "left_arm"
  Selector1/1 -> Gain/1
  DoFs converter1/4 -> "qjDot(t) "/4  "left_leg"
  DoFs converter1/5 -> "qjDot(t) "/5  "right_leg"
  DoFs converter1/3 -> "qjDot(t) "/3  "right_arm"
  DoFs converter1/1 -> "qjDot(t) "/1  "torso"
  DoFs converter1/2 -> "qjDot(t) "/2  "left_arm"
  nu/1 -> Selector1/1, Selector2/1
  Selector2/1 -> Demux/1
  Demux/1 -> linear and angular  base velocity/1  "vb"
  Demux/2 -> Gain1/1  "wb"
  Gain/1 -> DoFs converter1/1
  Gain1/1 -> linear and angular  base velocity/2

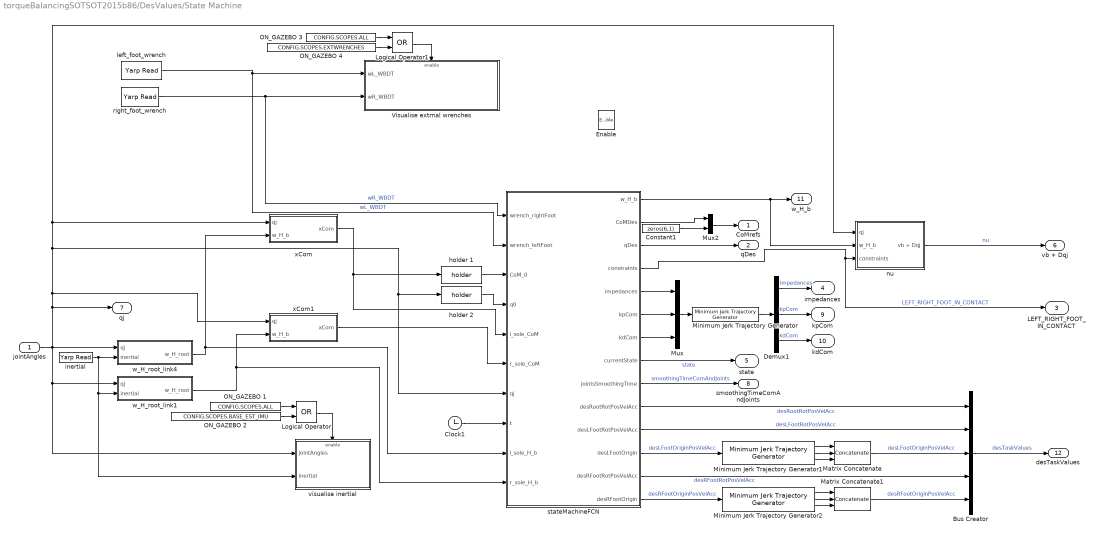
== system torqueBalancingSOTSOT2015b86/DesValues/State Machine ==
  jointAngles : Inport
  Enable : EnablePort
  Bus Creator : BusCreator  Inputs='desRootRotPosVelAcc','desLFootRotPosVelAcc','desLFootOriginPosVelAcc','desRFootRotPosVelAcc','desRFootOriginPosVelAcc'
  Clock1 : Clock
  Constant1 : Constant  Value=zeros(6,1)
  Demux1 : Demux  Outputs=[ROBOT_DOF,3,3]
  Logical Operator : Logic  Operator=OR  AllPortsSameDT=off  OutDataTypeStr=boolean
  Logical Operator1 : Logic  Operator=OR  AllPortsSameDT=off  OutDataTypeStr=boolean
  Matrix Concatenate : Concatenate  NumInputs=3  Mode=Multidimensional array  ConcatenateDimension=2
  Matrix Concatenate1 : Concatenate  NumInputs=3  Mode=Multidimensional array  ConcatenateDimension=2
  Minimum Jerk Trajectory Generator : WBToolboxLibrary/Utilities/Minimum Jerk Trajectory Generator  externalSettlingTime=off  settlingTime=gain.SmoothingTimeGainScheduling  sampleTime=CONFIG.Ts  resetOnSettlingTime=off  firstDerivatives=off  secondDerivatives=off  explicitInitialValue=off
  Minimum Jerk Trajectory Generator1 : WBToolboxLibrary/Utilities/Minimum Jerk Trajectory Generator  externalSettlingTime=off  settlingTime=gain.SmoothingTimeGainScheduling  sampleTime=CONFIG.Ts  resetOnSettlingTime=off  firstDerivatives=on  secondDerivatives=on  explicitInitialValue=off
  Minimum Jerk Trajectory Generator2 : WBToolboxLibrary/Utilities/Minimum Jerk Trajectory Generator  externalSettlingTime=off  settlingTime=gain.SmoothingTimeGainScheduling  sampleTime=CONFIG.Ts  resetOnSettlingTime=off  firstDerivatives=on  secondDerivatives=on  explicitInitialValue=off
  Mux : Mux  Inputs=3
  Mux2 : Mux  Inputs=2
  ON_GAZEBO 1 : Constant  Value=CONFIG.SCOPES.ALL
  ON_GAZEBO 2 : Constant  Value=CONFIG.SCOPES.BASE_EST_IMU
  ON_GAZEBO 3 : Constant  Value=CONFIG.SCOPES.ALL
  ON_GAZEBO 4 : Constant  Value=CONFIG.SCOPES.EXTWRENCHES
  "Visualise extrnal wrenches  " : Subsystem
  holder 1 : WBToolboxLibrary/Utilities/holder 
  holder 2 : WBToolboxLibrary/Utilities/holder 
  inertial : WBToolboxLibrary/Utilities/Yarp Read  portName=PORTS.IMU  signalSize=12  blocking=off  timestamp=off  autoconnect=on  errorOnConnection=on
  left_foot_wrench : WBToolboxLibrary/Utilities/Yarp Read  portName=PORTS.WBDT_LEFTLEG_EE  signalSize=6  blocking=off  timestamp=off  autoconnect=on  errorOnConnection=off
  nu : Subsystem
  right_foot_wrench : WBToolboxLibrary/Utilities/Yarp Read  portName=PORTS.WBDT_RIGHTLEG_EE  signalSize=6  blocking=off  timestamp=off  autoconnect=on  errorOnConnection=off
  stateMachineFCN : MATLAB Function  TreatAsAtomicUnit=on
      settings: PermitHierarchicalResolution=ParametersOnly
  visualise inertial : Subsystem
  w_H_root_link1 : Subsystem  mask{link_name='r_sole'}
      mask prompts: link_name "link name"
      mask help:
      | This block evaluates the homogeneous transformation between the world and the root link, i.e. ^wH_b. It assumes that the link specified by the variable 'link_name' has a constant position
      | w.r.t. an inertial frame, but it can rotate arbitrarily. This rotation is retrived from the IMU sensor.
      mask Display:
      | str = strrep(link_name, '_','\_');
      | port_label('output',1,['{}^{',str '}H_{root}'],'texmode','on')
      | clear str;
      | 
      | port_label('input',1,'q_j','texmode','on')
      | 
      | port_label('input',2,'inertial','texmode','on')
  w_H_root_link4 : Subsystem  mask{link_name='l_sole'}
      mask prompts: link_name "link name"
      mask help:
      | This block evaluates the homogeneous transformation between the world and the root link, i.e. ^wH_b. It assumes that the link specified by the variable 'link_name' has a constant position
      | w.r.t. an inertial frame, but it can rotate arbitrarily. This rotation is retrived from the IMU sensor.
      mask Display:
      | str = strrep(link_name, '_','\_');
      | port_label('output',1,['{}^{',str '}H_{root}'],'texmode','on')
      | clear str;
      | 
      | port_label('input',1,'q_j','texmode','on')
      | 
      | port_label('input',2,'inertial','texmode','on')
  xCom : Subsystem
  xCom1 : Subsystem
  CoMrefs : Outport
  qDes : Outport  Port=2
  LEFT_RIGHT_FOOT_IN_CONTACT : Outport  Port=3
  impedances : Outport  Port=4
  state : Outport  Port=5
  vb + Dqj : Outport  Port=6
  qj : Outport  Port=7
  smoothingTimeComAndJoints : Outport  Port=8
  kpCom : Outport  Port=9
  kdCom : Outport  Port=10
  w_H_b : Outport  Port=11
  desTaskValues : Outport  Port=12
  wires:
  right_foot_wrench/1 -> "Visualise extrnal wrenches  "/2(wR_WBDT), stateMachineFCN/1(wrench_rightFoot)  "wR_WBDT"
  xCom/1(xCom) -> stateMachineFCN/5(l_sole_CoM), holder 1/1
  holder 1/1 -> stateMachineFCN/3(CoM_0)
  holder 2/1 -> stateMachineFCN/4(q0)
  Clock1/1 -> stateMachineFCN/8(t)
  stateMachineFCN/3(qDes) -> qDes/1
  stateMachineFCN/2(CoMDes) -> Mux2/1
  Mux2/1 -> CoMrefs/1
  Constant1/1 -> Mux2/2
  stateMachineFCN/8(currentState) -> state/1  "state"
  stateMachineFCN/4(constraints) -> LEFT_RIGHT_FOOT_IN_CONTACT/1, nu/3("constraints ")  "LEFT_RIGHT_FOOT_IN_CONTACT"
  left_foot_wrench/1 -> "Visualise extrnal wrenches  "/1(wL_WBDT), stateMachineFCN/2(wrench_leftFoot)  "wL_WBDT"
  stateMachineFCN/1(w_H_b) -> w_H_b/1, nu/2(w_H_b)
  xCom1/1(xCom) -> stateMachineFCN/6(r_sole_CoM)
  nu/1(vb + Dqj) -> vb + Dqj/1  "nu"
  w_H_root_link4/1(w_H_root) -> stateMachineFCN/9(l_sole_H_b), xCom/2(w_H_b)
  w_H_root_link1/1(w_H_root) -> stateMachineFCN/10(r_sole_H_b), xCom1/2(w_H_b)
  jointAngles/1 -> w_H_root_link4/1(qj), w_H_root_link1/1(qj), visualise inertial/1(jointAngles), nu/1(qj), xCom/1(qj), stateMachineFCN/7(qj), holder 2/1, xCom1/1(qj), qj/1
  inertial/1 -> w_H_root_link1/2(inertial), visualise inertial/2(inertial), w_H_root_link4/2(inertial)
  stateMachineFCN/9(jointsSmoothingTime) -> smoothingTimeComAndJoints/1  "smoothingTimeComAndJoints"
  Logical Operator1/1 -> "Visualise extrnal wrenches  "/Enable
  ON_GAZEBO 1/1 -> Logical Operator/1
  ON_GAZEBO 2/1 -> Logical Operator/2
  Logical Operator/1 -> visualise inertial/Enable
  ON_GAZEBO 3/1 -> Logical Operator1/1
  ON_GAZEBO 4/1 -> Logical Operator1/2
  stateMachineFCN/6(kpCom) -> Mux/2
  Demux1/3 -> kdCom/1  "kdCom"
  stateMachineFCN/7(kdCom) -> Mux/3
  stateMachineFCN/5(impedances) -> Mux/1
  Mux/1 -> Minimum Jerk Trajectory Generator/1
  Minimum Jerk Trajectory Generator/1 -> Demux1/1
  Demux1/1 -> impedances/1  "impedances"
  Demux1/2 -> kpCom/1  "kpCom"
  stateMachineFCN/11(desLFootRotPosVelAcc) -> Bus Creator/2  "desLFootRotPosVelAcc"
  stateMachineFCN/13(desRFootRotPosVelAcc) -> Bus Creator/4  "desRFootRotPosVelAcc"
  Matrix Concatenate/1 -> Bus Creator/3  "desLFootOriginPosVelAcc"
  stateMachineFCN/10(desRootRotPosVelAcc) -> Bus Creator/1  "desRootRotPosVelAcc"
  Bus Creator/1 -> desTaskValues/1  "desTaskValues"
  Matrix Concatenate1/1 -> Bus Creator/5  "desRFootOriginPosVelAcc"
  stateMachineFCN/12(desLFootOrigin) -> Minimum Jerk Trajectory Generator1/1  "desLFootOriginPosVelAcc"
  stateMachineFCN/14(desRFootOrigin) -> Minimum Jerk Trajectory Generator2/1  "desRFootOriginPosVelAcc"
  Minimum Jerk Trajectory Generator1/1 -> Matrix Concatenate/1
  Minimum Jerk Trajectory Generator1/2 -> Matrix Concatenate/2
  Minimum Jerk Trajectory Generator1/3 -> Matrix Concatenate/3
  Minimum Jerk Trajectory Generator2/1 -> Matrix Concatenate1/1
  Minimum Jerk Trajectory Generator2/2 -> Matrix Concatenate1/2
  Minimum Jerk Trajectory Generator2/3 -> Matrix Concatenate1/3

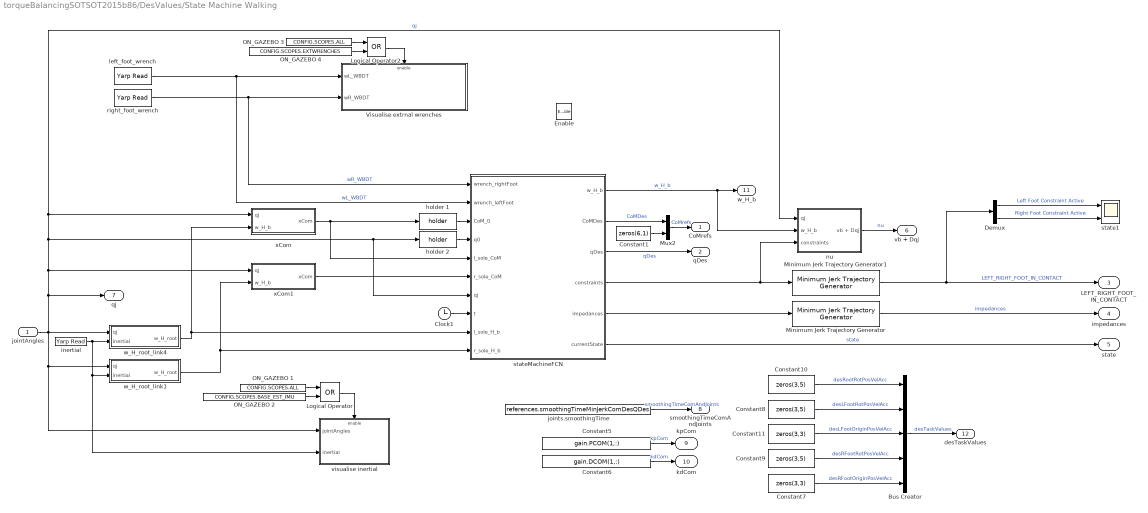
== system torqueBalancingSOTSOT2015b86/DesValues/State Machine Walking ==
  jointAngles : Inport
  Enable : EnablePort
  Bus Creator : BusCreator  Inputs='desRootRotPosVelAcc','desLFootRotPosVelAcc','desLFootOriginPosVelAcc','desRFootRotPosVelAcc','desRFootOriginPosVelAcc'
  Clock1 : Clock
  Constant1 : Constant  Value=zeros(6,1)
  Constant10 : Constant  Value=zeros(3,5)
  Constant11 : Constant  Value=zeros(3,3)
  Constant5 : Constant  Value=gain.PCOM(1,:)
  Constant6 : Constant  Value=gain.DCOM(1,:)
  Constant7 : Constant  Value=zeros(3,3)
  Constant8 : Constant  Value=zeros(3,5)
  Constant9 : Constant  Value=zeros(3,5)
  Demux : Demux  Outputs=2
  Logical Operator : Logic  Operator=OR  AllPortsSameDT=off  OutDataTypeStr=boolean
  Logical Operator2 : Logic  Operator=OR  AllPortsSameDT=off  OutDataTypeStr=boolean
  Minimum Jerk Trajectory Generator : WBToolboxLibrary/Utilities/Minimum Jerk Trajectory Generator  externalSettlingTime=off  settlingTime=gain.SmoothingTimeImp  sampleTime=CONFIG.Ts  resetOnSettlingTime=off  firstDerivatives=off  secondDerivatives=off  explicitInitialValue=off
  Minimum Jerk Trajectory Generator1 : WBToolboxLibrary/Utilities/Minimum Jerk Trajectory Generator  externalSettlingTime=off  settlingTime=CONFIG.smoothingTimeTranDynamics  sampleTime=CONFIG.Ts  resetOnSettlingTime=off  firstDerivatives=off  secondDerivatives=off  explicitInitialValue=off
  Mux2 : Mux  Inputs=2
  ON_GAZEBO 1 : Constant  Value=CONFIG.SCOPES.ALL
  ON_GAZEBO 2 : Constant  Value=CONFIG.SCOPES.BASE_EST_IMU
  ON_GAZEBO 3 : Constant  Value=CONFIG.SCOPES.ALL
  ON_GAZEBO 4 : Constant  Value=CONFIG.SCOPES.EXTWRENCHES
  "Visualise extrnal wrenches  " : Subsystem
  holder 1 : WBToolboxLibrary/Utilities/holder 
  holder 2 : WBToolboxLibrary/Utilities/holder 
  inertial : WBToolboxLibrary/Utilities/Yarp Read  portName=PORTS.IMU  signalSize=12  blocking=off  timestamp=off  autoconnect=on  errorOnConnection=on
  joints.smoothingTime : Constant  Value=references.smoothingTimeMinJerkComDesQDes
  left_foot_wrench : WBToolboxLibrary/Utilities/Yarp Read  portName=PORTS.WBDT_LEFTLEG_EE  signalSize=6  blocking=off  timestamp=off  autoconnect=on  errorOnConnection=off
  nu : Subsystem
  right_foot_wrench : WBToolboxLibrary/Utilities/Yarp Read  portName=PORTS.WBDT_RIGHTLEG_EE  signalSize=6  blocking=off  timestamp=off  autoconnect=on  errorOnConnection=off
  state1 : Scope  NumInputPorts=2
  stateMachineFCN : MATLAB Function  Priority=-1  TreatAsAtomicUnit=on
      settings: PermitHierarchicalResolution=ParametersOnly
  visualise inertial : Subsystem
  w_H_root_link1 : Subsystem  mask{link_name='r_sole'}
      mask prompts: link_name "link name"
      mask help:
      | This block evaluates the homogeneous transformation between the world and the root link, i.e. ^wH_b. It assumes that the link specified by the variable 'link_name' has a constant position
      | w.r.t. an inertial frame, but it can rotate arbitrarily. This rotation is retrived from the IMU sensor.
      mask Display:
      | str = strrep(link_name, '_','\_');
      | port_label('output',1,['{}^{',str '}H_{root}'],'texmode','on')
      | clear str;
      | 
      | port_label('input',1,'q_j','texmode','on')
      | 
      | port_label('input',2,'inertial','texmode','on')
  w_H_root_link4 : Subsystem  mask{link_name='l_sole'}
      mask prompts: link_name "link name"
      mask help:
      | This block evaluates the homogeneous transformation between the world and the root link, i.e. ^wH_b. It assumes that the link specified by the variable 'link_name' has a constant position
      | w.r.t. an inertial frame, but it can rotate arbitrarily. This rotation is retrived from the IMU sensor.
      mask Display:
      | str = strrep(link_name, '_','\_');
      | port_label('output',1,['{}^{',str '}H_{root}'],'texmode','on')
      | clear str;
      | 
      | port_label('input',1,'q_j','texmode','on')
      | 
      | port_label('input',2,'inertial','texmode','on')
  xCom : Subsystem
  xCom1 : Subsystem
  CoMrefs : Outport
  qDes : Outport  Port=2
  LEFT_RIGHT_FOOT_IN_CONTACT : Outport  Port=3
  impedances : Outport  Port=4
  state : Outport  Port=5
  vb + Dqj : Outport  Port=6
  qj : Outport  Port=7
  smoothingTimeComAndJoints : Outport  Port=8
  kpCom : Outport  Port=9
  kdCom : Outport  Port=10
  w_H_b : Outport  Port=11
  desTaskValues : Outport  Port=12
  wires:
  stateMachineFCN/3(qDes) -> qDes/1  "qDes"
  stateMachineFCN/2(CoMDes) -> Mux2/1  "CoMDes"
  Mux2/1 -> CoMrefs/1  "CoMrefs"
  Constant1/1 -> Mux2/2
  stateMachineFCN/5(impedances) -> Minimum Jerk Trajectory Generator/1
  stateMachineFCN/6(currentState) -> state/1  "state"
  Minimum Jerk Trajectory Generator1/1 -> Demux/1, LEFT_RIGHT_FOOT_IN_CONTACT/1  "LEFT_RIGHT_FOOT_IN_CONTACT"
  stateMachineFCN/4(constraints) -> nu/3("constraints "), Minimum Jerk Trajectory Generator1/1
  Demux/1 -> state1/1  "Left Foot Constraint Active"
  Demux/2 -> state1/2  "Right Foot Constraint Active"
  stateMachineFCN/1(w_H_b) -> nu/2(w_H_b), w_H_b/1  "w_H_b"
  nu/1(vb + Dqj) -> vb + Dqj/1  "nu"
  Minimum Jerk Trajectory Generator/1 -> impedances/1  "impedances"
  joints.smoothingTime/1 -> smoothingTimeComAndJoints/1  "smoothingTimeComAndJoints"
  Constant5/1 -> kpCom/1  "kpCom"
  Constant6/1 -> kdCom/1  "kdCom"
  Constant8/1 -> Bus Creator/2  "desLFootRotPosVelAcc"
  Constant9/1 -> Bus Creator/4  "desRFootRotPosVelAcc"
  Constant11/1 -> Bus Creator/3  "desLFootOriginPosVelAcc"
  Constant10/1 -> Bus Creator/1  "desRootRotPosVelAcc"
  Bus Creator/1 -> desTaskValues/1  "desTaskValues"
  Constant7/1 -> Bus Creator/5  "desRFootOriginPosVelAcc"
  right_foot_wrench/1 -> stateMachineFCN/1(wrench_rightFoot), "Visualise extrnal wrenches  "/2(wR_WBDT)  "wR_WBDT"
  xCom/1(xCom) -> stateMachineFCN/5(l_sole_CoM), holder 1/1
  holder 1/1 -> stateMachineFCN/3(CoM_0)
  holder 2/1 -> stateMachineFCN/4(q0)
  Clock1/1 -> stateMachineFCN/8(t)
  left_foot_wrench/1 -> stateMachineFCN/2(wrench_leftFoot), "Visualise extrnal wrenches  "/1(wL_WBDT)  "wL_WBDT"
  xCom1/1(xCom) -> stateMachineFCN/6(r_sole_CoM)
  w_H_root_link4/1(w_H_root) -> stateMachineFCN/9(l_sole_H_b), xCom/2(w_H_b)
  w_H_root_link1/1(w_H_root) -> stateMachineFCN/10(r_sole_H_b), xCom1/2(w_H_b)
  jointAngles/1 -> w_H_root_link4/1(qj), w_H_root_link1/1(qj), visualise inertial/1(jointAngles), nu/1(qj), xCom/1(qj), stateMachineFCN/7(qj), holder 2/1, xCom1/1(qj), qj/1  "qj"
  inertial/1 -> w_H_root_link1/2(inertial), visualise inertial/2(inertial), w_H_root_link4/2(inertial)
  Logical Operator2/1 -> "Visualise extrnal wrenches  "/Enable
  ON_GAZEBO 1/1 -> Logical Operator/1
  ON_GAZEBO 2/1 -> Logical Operator/2
  Logical Operator/1 -> visualise inertial/Enable
  ON_GAZEBO 3/1 -> Logical Operator2/1
  ON_GAZEBO 4/1 -> Logical Operator2/2

== system torqueBalancingSOTSOT2015b86/Dump and visualize/ZMPs ==
  fDesQP : Inport
  Demux1 : Demux  Outputs=3
  Demux2 : Demux  Outputs=3
  Divide{4..7} (4 alike) : Product  Inputs=*/
  Gain3 : Gain  Gain=-1
  Gain4 : Gain  Gain=-1
  Mux : Mux  Inputs=2
  Mux1 : Mux  Inputs=2
  fz taux tauy Left : Selector  InputPortWidth=12  IndexOptions=Index vector (dialog)  Indices=[3 4 5]  OutputSizes=1
  fz taux tauy Right : Selector  InputPortWidth=12  IndexOptions=Index vector (dialog)  Indices=[9 10 11]  OutputSizes=1
  ZMP_LeftFoot : Outport
  ZMP_RightFoot : Outport  Port=2
  wires:
  fz taux tauy Left/1 -> Demux1/1
  Demux1/1 -> Divide4/2, Divide5/2
  Divide7/1 -> Gain4/1
  Divide4/1 -> Mux/2
  Divide5/1 -> Gain3/1
  fz taux tauy Right/1 -> Demux2/1
  Demux2/1 -> Divide6/2, Divide7/2
  fDesQP/1 -> fz taux tauy Left/1, fz taux tauy Right/1
  Gain3/1 -> Mux/1
  Mux/1 -> ZMP_LeftFoot/1
  Divide6/1 -> Mux1/2
  Gain4/1 -> Mux1/1
  Mux1/1 -> ZMP_RightFoot/1
  Demux1/2 -> Divide4/1  "tauxL"
  Demux1/3 -> Divide5/1  "tauyL"
  Demux2/2 -> Divide6/1  "tauxR"
  Demux2/3 -> Divide7/1  "tauyR"

== system torqueBalancingSOTSOT2015b86/Dump and visualize/plotNorms ==
  qTile_LeftLeg : Inport
  qTile_RightLeg : Inport  Port=2
  state : Inport  Port=3
  Constant : Constant  Value=sm.joints.thresholdInContact
  Constant2 : Constant  Value=sm.joints.thresholdNotInContact
  Mux : Mux  Inputs=3
  Mux1 : Mux  Inputs=3
  norm : MATLAB Function  TreatAsAtomicUnit=on
      settings: PermitHierarchicalResolution=ParametersOnly
  norm(qTilde) : Scope  NumInputPorts=3
  norm1 : MATLAB Function  TreatAsAtomicUnit=on
      settings: PermitHierarchicalResolution=ParametersOnly
  wires:
  Constant/1 -> Mux1/2, Mux/2  "thresholdInContact"
  qTile_LeftLeg/1 -> norm1/1(u)
  qTile_RightLeg/1 -> norm/1(u)
  norm/1(normU) -> Mux1/1  "norm(qTilde_RightL)"
  norm1/1(normU) -> Mux/1  "norm(qTilde_LeftL)"
  Mux/1 -> norm(qTilde)/1
  Mux1/1 -> norm(qTilde)/2
  Constant2/1 -> Mux1/3, Mux/3  "thresholdNotInContact"
  state/1 -> norm(qTilde)/3
